simulink model "CW_M107"  (R2017b)
settings: Solver=VariableStepAuto  StartTime=0.0  StopTime=10.0  RelTol=1e-3
undefined symbols (not defined in the file): b, J, K, L, R

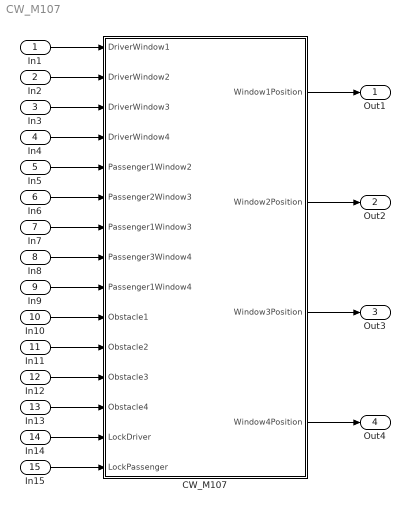
== system CW_M107 ==
  In1 : Inport
  In2 : Inport  Port=2
  In3 : Inport  Port=3
  In4 : Inport  Port=4
  In5 : Inport  Port=5
  In6 : Inport  Port=6
  In7 : Inport  Port=7
  In8 : Inport  Port=8
  In9 : Inport  Port=9
  In10 : Inport  Port=10
  In11 : Inport  Port=11
  In12 : Inport  Port=12
  In13 : Inport  Port=13
  In14 : Inport  Port=14
  In15 : Inport  Port=15
  CW_M107 : Subsystem
  Out1 : Outport
  Out2 : Outport  Port=2
  Out3 : Outport  Port=3
  Out4 : Outport  Port=4
  wires:
  In13/1 -> CW_M107/13(Obstacle4)
  In6/1 -> CW_M107/6(Passenger2Window3)
  CW_M107/2(Window2Position) -> Out2/1
  In9/1 -> CW_M107/9(Passenger1Window4)
  In7/1 -> CW_M107/7(Passenger1Window3)
  In1/1 -> CW_M107/1(DriverWindow1)
  CW_M107/3(Window3Position) -> Out3/1
  In3/1 -> CW_M107/3(DriverWindow3)
  In8/1 -> CW_M107/8(Passenger3Window4)
  CW_M107/4(Window4Position) -> Out4/1
  In15/1 -> CW_M107/15(LockPassenger)
  In5/1 -> CW_M107/5(Passenger1Window2)
  In4/1 -> CW_M107/4(DriverWindow4)
  In10/1 -> CW_M107/10(Obstacle1)
  In14/1 -> CW_M107/14(LockDriver)
  In11/1 -> CW_M107/11(Obstacle2)
  In12/1 -> CW_M107/12(Obstacle3)
  In2/1 -> CW_M107/2(DriverWindow2)
  CW_M107/1(Window1Position) -> Out1/1

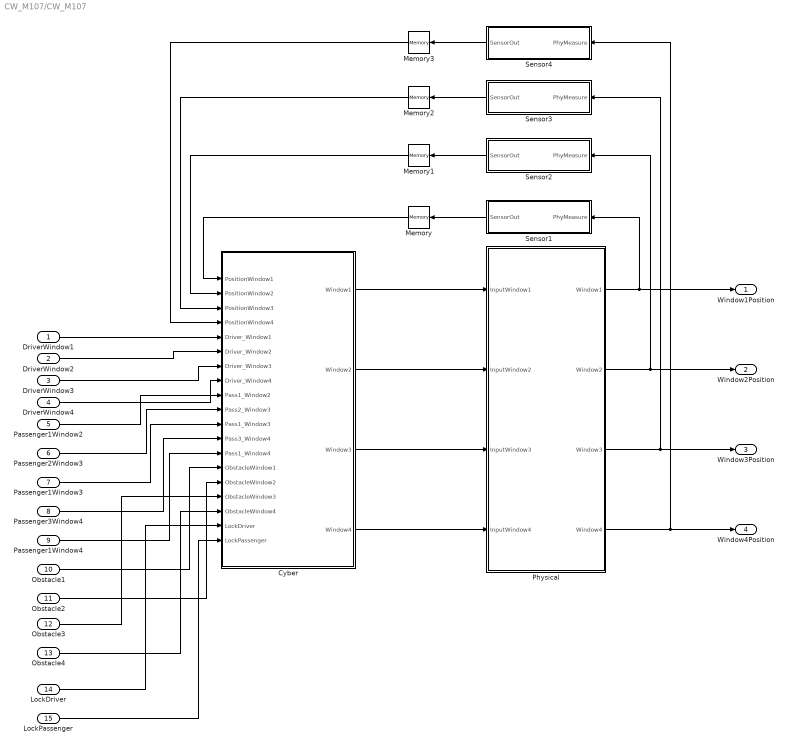
== system CW_M107/CW_M107 ==
  DriverWindow1 : Inport
  DriverWindow2 : Inport  Port=2
  DriverWindow3 : Inport  Port=3
  DriverWindow4 : Inport  Port=4
  Passenger1Window2 : Inport  Port=5
  Passenger2Window3 : Inport  Port=6
  Passenger1Window3 : Inport  Port=7
  Passenger3Window4 : Inport  Port=8
  Passenger1Window4 : Inport  Port=9
  Obstacle1 : Inport  Port=10
  Obstacle2 : Inport  Port=11
  Obstacle3 : Inport  Port=12
  Obstacle4 : Inport  Port=13
  LockDriver : Inport  Port=14
  LockPassenger : Inport  Port=15
  Cyber : Subsystem
  Memory{,1..3} (4 alike) : Memory
  Physical : Subsystem
  Sensor1 : Subsystem
  Sensor2 : Subsystem
  Sensor3 : Subsystem
  Sensor4 : Subsystem
  Window1Position : Outport
  Window2Position : Outport  Port=2
  Window3Position : Outport  Port=3
  Window4Position : Outport  Port=4
  wires:
  LockPassenger/1 -> Cyber/19(LockPassenger)
  LockDriver/1 -> Cyber/18(LockDriver)
  Obstacle4/1 -> Cyber/17(ObstacleWindow4)
  Obstacle3/1 -> Cyber/16(ObstacleWindow3)
  Obstacle2/1 -> Cyber/15(ObstacleWindow2)
  Passenger1Window4/1 -> Cyber/13(Pass1_Window4)
  Passenger3Window4/1 -> Cyber/12(Pass3_Window4)
  Passenger1Window3/1 -> Cyber/11(Pass1_Window3)
  Passenger2Window3/1 -> Cyber/10(Pass2_Window3)
  Passenger1Window2/1 -> Cyber/9(Pass1_Window2)
  DriverWindow4/1 -> Cyber/8(Driver_Window4)
  DriverWindow3/1 -> Cyber/7(Driver_Window3)
  DriverWindow1/1 -> Cyber/5(Driver_Window1)
  DriverWindow2/1 -> Cyber/6(Driver_Window2)
  Sensor1/1(SensorOut) -> Memory/1
  Sensor2/1(SensorOut) -> Memory1/1
  Sensor3/1(SensorOut) -> Memory2/1
  Sensor4/1(SensorOut) -> Memory3/1
  Obstacle1/1 -> Cyber/14(ObstacleWindow1)
  Memory3/1 -> Cyber/4(PositionWindow4)
  Memory2/1 -> Cyber/3(PositionWindow3)
  Memory1/1 -> Cyber/2(PositionWindow2)
  Memory/1 -> Cyber/1(PositionWindow1)
  Physical/4(Window4) -> Window4Position/1, Sensor4/1(PhyMeasure)
  Physical/3(Window3) -> Sensor3/1(PhyMeasure), Window3Position/1
  Physical/2(Window2) -> Window2Position/1, Sensor2/1(PhyMeasure)
  Physical/1(Window1) -> Window1Position/1, Sensor1/1(PhyMeasure)
  Cyber/1(Window1) -> Physical/1(InputWindow1)
  Cyber/2(Window2) -> Physical/2(InputWindow2)
  Cyber/3(Window3) -> Physical/3(InputWindow3)
  Cyber/4(Window4) -> Physical/4(InputWindow4)

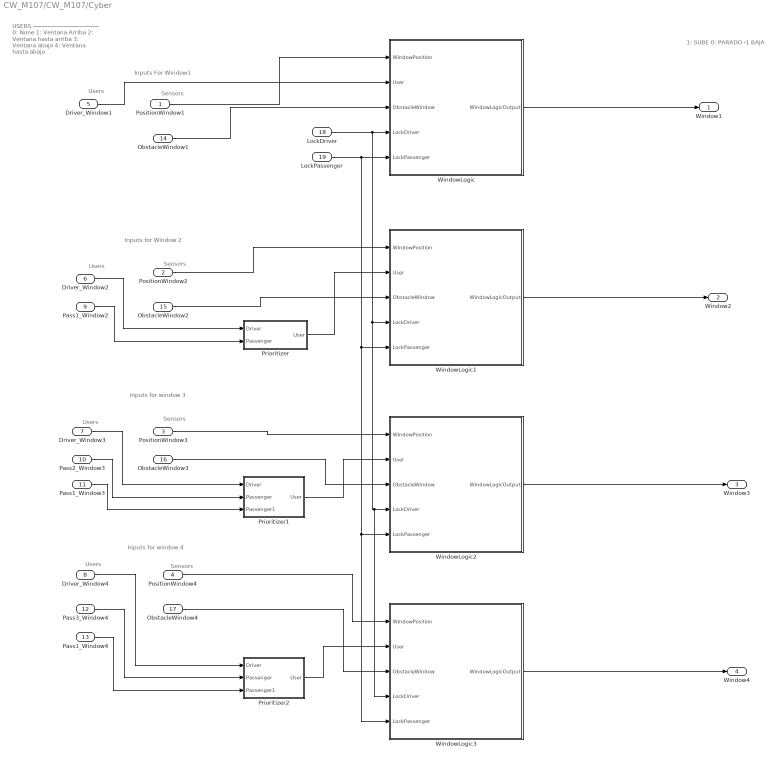
== system CW_M107/CW_M107/Cyber ==
  note: Inputs For Window1
  note: Inputs for Window 2
  note: Inputs for window 3
  note: Inputs for window 4
  note: Sensors
  note: Users
  note: Users
  note: Sensors
  note: Users
  note: Sensors
  note: Users
  note: Sensors
  note: USERS
      | ---------------------------------
      | 0: None
      | 1: Ventana Arriba
      | 2: Ventana hasta arriba
      | 3: Ventana abajo
      | 4: Ventana hasta abajo
  note: 1: SUBE
      | 0: PARADO
      | -1 BAJA
  PositionWindow1 : Inport
  PositionWindow2 : Inport  Port=2
  PositionWindow3 : Inport  Port=3
  PositionWindow4 : Inport  Port=4
  Driver_Window1 : Inport  Port=5
  Driver_Window2 : Inport  Port=6
  Driver_Window3 : Inport  Port=7
  Driver_Window4 : Inport  Port=8
  Pass1_Window2 : Inport  Port=9
  Pass2_Window3 : Inport  Port=10
  Pass1_Window3 : Inport  Port=11
  Pass3_Window4 : Inport  Port=12
  Pass1_Window4 : Inport  Port=13
  ObstacleWindow1 : Inport  Port=14
  ObstacleWindow2 : Inport  Port=15
  ObstacleWindow3 : Inport  Port=16
  ObstacleWindow4 : Inport  Port=17
  LockDriver : Inport  Port=18
  LockPassenger : Inport  Port=19
  Prioritizer : Subsystem
  Prioritizer1 : Subsystem
  Prioritizer2 : Subsystem
  WindowLogic : Subsystem
  WindowLogic1 : Subsystem
  WindowLogic2 : Subsystem
  WindowLogic3 : Subsystem
  Window1 : Outport
  Window2 : Outport  Port=2
  Window3 : Outport  Port=3
  Window4 : Outport  Port=4
  wires:
  WindowLogic3/1(WindowLogicOutput) -> Window4/1
  WindowLogic2/1(WindowLogicOutput) -> Window3/1
  Prioritizer2/1(User) -> WindowLogic3/2(User)
  ObstacleWindow4/1 -> WindowLogic3/3(ObstacleWindow)
  PositionWindow4/1 -> WindowLogic3/1(WindowPosition)
  Pass1_Window4/1 -> Prioritizer2/3(Passenger1)
  Pass3_Window4/1 -> Prioritizer2/2(Passenger)
  Driver_Window4/1 -> Prioritizer2/1(Driver)
  Pass1_Window3/1 -> Prioritizer1/3(Passenger1)
  Pass2_Window3/1 -> Prioritizer1/2(Passenger)
  Driver_Window3/1 -> Prioritizer1/1(Driver)
  ObstacleWindow3/1 -> WindowLogic2/3(ObstacleWindow)
  PositionWindow3/1 -> WindowLogic2/1(WindowPosition)
  Prioritizer1/1(User) -> WindowLogic2/2(User)
  WindowLogic1/1(WindowLogicOutput) -> Window2/1
  ObstacleWindow2/1 -> WindowLogic1/3(ObstacleWindow)
  PositionWindow2/1 -> WindowLogic1/1(WindowPosition)
  Pass1_Window2/1 -> Prioritizer/2(Passenger)
  Driver_Window2/1 -> Prioritizer/1(Driver)
  Prioritizer/1(User) -> WindowLogic1/2(User)
  WindowLogic/1(WindowLogicOutput) -> Window1/1
  Driver_Window1/1 -> WindowLogic/2(User)
  ObstacleWindow1/1 -> WindowLogic/3(ObstacleWindow)
  PositionWindow1/1 -> WindowLogic/1(WindowPosition)
  LockPassenger/1 -> WindowLogic/5(LockPassenger), WindowLogic2/5(LockPassenger), WindowLogic3/5(LockPassenger), WindowLogic1/5(LockPassenger)
  LockDriver/1 -> WindowLogic/4(LockDriver), WindowLogic2/4(LockDriver), WindowLogic3/4(LockDriver), WindowLogic1/4(LockDriver)

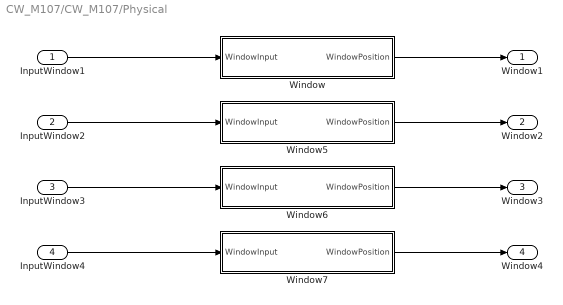
== system CW_M107/CW_M107/Physical ==
  InputWindow1 : Inport
  InputWindow2 : Inport  Port=2
  InputWindow3 : Inport  Port=3
  InputWindow4 : Inport  Port=4
  Window : Subsystem
  Window5 : Subsystem
  Window6 : Subsystem
  Window7 : Subsystem
  Window1 : Outport
  Window2 : Outport  Port=2
  Window3 : Outport  Port=3
  Window4 : Outport  Port=4
  wires:
  Window7/1(WindowPosition) -> Window4/1
  Window6/1(WindowPosition) -> Window3/1
  Window5/1(WindowPosition) -> Window2/1
  Window/1(WindowPosition) -> Window1/1
  InputWindow4/1 -> Window7/1(WindowInput)
  InputWindow3/1 -> Window6/1(WindowInput)
  InputWindow2/1 -> Window5/1(WindowInput)
  InputWindow1/1 -> Window/1(WindowInput)

== system CW_M107/CW_M107/Sensor1 ==
  PhyMeasure : Inport
  SensorOut : Outport
  wires:
  PhyMeasure/1 -> SensorOut/1

== system CW_M107/CW_M107/Sensor2 ==
  PhyMeasure : Inport
  SensorOut : Outport
  wires:
  PhyMeasure/1 -> SensorOut/1

== system CW_M107/CW_M107/Sensor3 ==
  PhyMeasure : Inport
  SensorOut : Outport
  wires:
  PhyMeasure/1 -> SensorOut/1

== system CW_M107/CW_M107/Sensor4 ==
  PhyMeasure : Inport
  SensorOut : Outport
  wires:
  PhyMeasure/1 -> SensorOut/1

== system CW_M107/CW_M107/Cyber/Prioritizer ==
  Driver : Inport
  Passenger : Inport  Port=2
  Switch : Switch  Criteria=u2 ~= 0
  User : Outport
  wires:
  Switch/1 -> User/1
  Passenger/1 -> Switch/3
  Driver/1 -> Switch/2, Switch/1

== system CW_M107/CW_M107/Cyber/Prioritizer1 ==
  Driver : Inport
  Passenger : Inport  Port=2
  Passenger1 : Inport  Port=3
  Switch : Switch  Criteria=u2 ~= 0
  Switch1 : Switch  Criteria=u2 ~= 0
  User : Outport
  wires:
  Switch1/1 -> Switch/3
  Passenger1/1 -> Switch1/3
  Driver/1 -> Switch/2, Switch/1
  Passenger/1 -> Switch1/2, Switch1/1
  Switch/1 -> User/1

== system CW_M107/CW_M107/Cyber/Prioritizer2 ==
  Driver : Inport
  Passenger : Inport  Port=2
  Passenger1 : Inport  Port=3
  Switch : Switch  Criteria=u2 ~= 0
  Switch1 : Switch  Criteria=u2 ~= 0
  User : Outport
  wires:
  Switch/1 -> User/1
  Passenger/1 -> Switch1/1, Switch1/2
  Driver/1 -> Switch/1, Switch/2
  Passenger1/1 -> Switch1/3
  Switch1/1 -> Switch/3

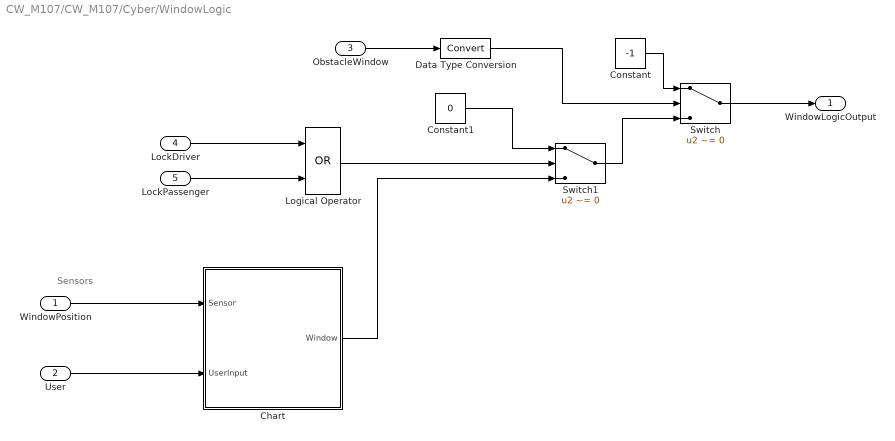
== system CW_M107/CW_M107/Cyber/WindowLogic ==
  note: Sensors
  WindowPosition : Inport
  User : Inport  Port=2
  ObstacleWindow : Inport  Port=3
  LockDriver : Inport  Port=4
  LockPassenger : Inport  Port=5
  Chart : Stateflow chart  TreatAsAtomicUnit=on
  Constant : Constant  Value=-1
  Constant1 : Constant  Value=0
  Data Type Conversion : DataTypeConversion
  Logical Operator : Logic  Operator=OR  AllPortsSameDT=off  OutDataTypeStr=boolean
  Switch : Switch  Criteria=u2 ~= 0  Threshold=1  ZeroCross=off
  Switch1 : Switch  Criteria=u2 ~= 0
  WindowLogicOutput : Outport
  wires:
  Logical Operator/1 -> Switch1/2
  Data Type Conversion/1 -> Switch/2
  Constant/1 -> Switch/1
  Chart/1(Window) -> Switch1/3
  User/1 -> Chart/2(UserInput)
  WindowPosition/1 -> Chart/1(Sensor)
  Switch1/1 -> Switch/3
  Constant1/1 -> Switch1/1
  Switch/1 -> WindowLogicOutput/1
  ObstacleWindow/1 -> Data Type Conversion/1
  LockPassenger/1 -> Logical Operator/2
  LockDriver/1 -> Logical Operator/1

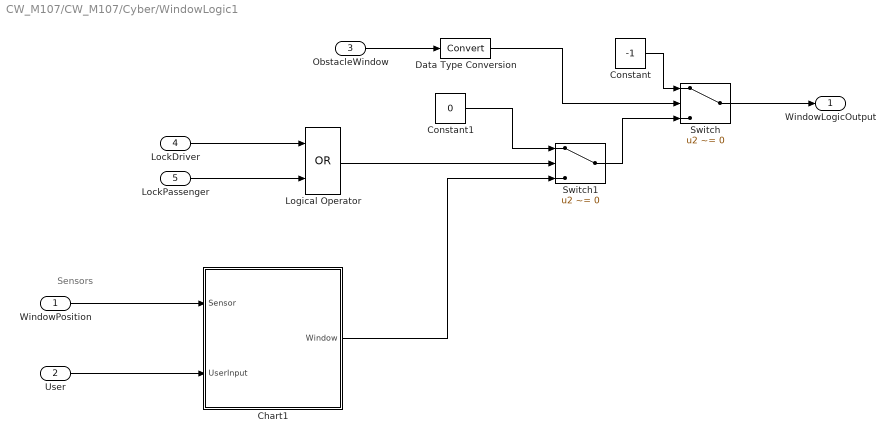
== system CW_M107/CW_M107/Cyber/WindowLogic1 ==
  note: Sensors
  WindowPosition : Inport
  User : Inport  Port=2
  ObstacleWindow : Inport  Port=3
  LockDriver : Inport  Port=4
  LockPassenger : Inport  Port=5
  Chart1 : Stateflow chart  TreatAsAtomicUnit=on
  Constant : Constant  Value=-1
  Constant1 : Constant  Value=0
  Data Type Conversion : DataTypeConversion
  Logical Operator : Logic  Operator=OR  AllPortsSameDT=off  OutDataTypeStr=boolean
  Switch : Switch  Criteria=u2 ~= 0  Threshold=1  ZeroCross=off
  Switch1 : Switch  Criteria=u2 ~= 0
  WindowLogicOutput : Outport
  wires:
  LockDriver/1 -> Logical Operator/1
  LockPassenger/1 -> Logical Operator/2
  ObstacleWindow/1 -> Data Type Conversion/1
  Switch/1 -> WindowLogicOutput/1
  Constant1/1 -> Switch1/1
  Switch1/1 -> Switch/3
  WindowPosition/1 -> Chart1/1(Sensor)
  User/1 -> Chart1/2(UserInput)
  Chart1/1(Window) -> Switch1/3
  Constant/1 -> Switch/1
  Data Type Conversion/1 -> Switch/2
  Logical Operator/1 -> Switch1/2

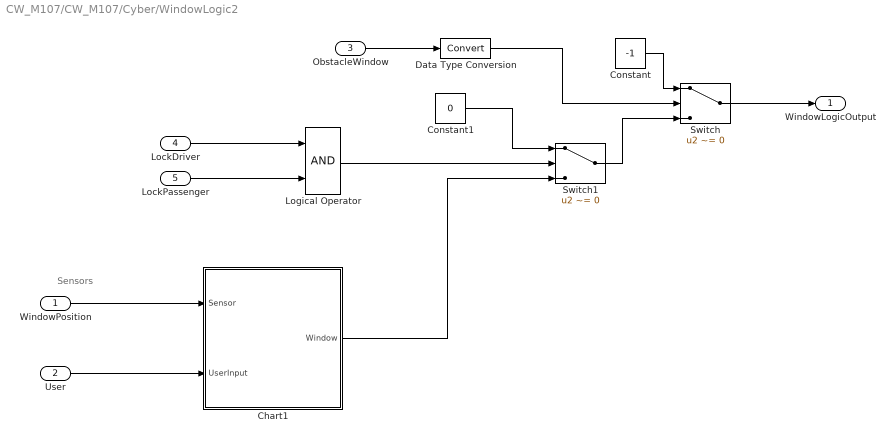
== system CW_M107/CW_M107/Cyber/WindowLogic2 ==
  note: Sensors
  WindowPosition : Inport
  User : Inport  Port=2
  ObstacleWindow : Inport  Port=3
  LockDriver : Inport  Port=4
  LockPassenger : Inport  Port=5
  Chart1 : Stateflow chart  TreatAsAtomicUnit=on
  Constant : Constant  Value=-1
  Constant1 : Constant  Value=0
  Data Type Conversion : DataTypeConversion
  Logical Operator : Logic  AllPortsSameDT=off  OutDataTypeStr=boolean
  Switch : Switch  Criteria=u2 ~= 0  Threshold=1  ZeroCross=off
  Switch1 : Switch  Criteria=u2 ~= 0
  WindowLogicOutput : Outport
  wires:
  Logical Operator/1 -> Switch1/2
  Data Type Conversion/1 -> Switch/2
  Constant/1 -> Switch/1
  Chart1/1(Window) -> Switch1/3
  User/1 -> Chart1/2(UserInput)
  WindowPosition/1 -> Chart1/1(Sensor)
  Switch1/1 -> Switch/3
  Constant1/1 -> Switch1/1
  Switch/1 -> WindowLogicOutput/1
  ObstacleWindow/1 -> Data Type Conversion/1
  LockPassenger/1 -> Logical Operator/2
  LockDriver/1 -> Logical Operator/1

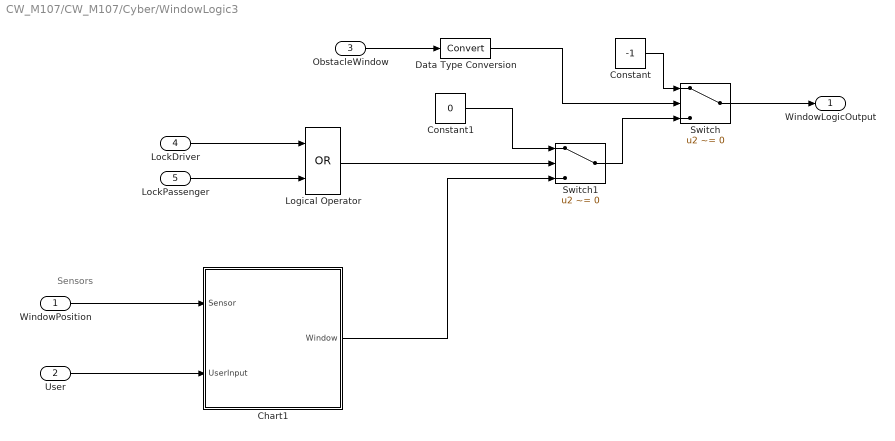
== system CW_M107/CW_M107/Cyber/WindowLogic3 ==
  note: Sensors
  WindowPosition : Inport
  User : Inport  Port=2
  ObstacleWindow : Inport  Port=3
  LockDriver : Inport  Port=4
  LockPassenger : Inport  Port=5
  Chart1 : Stateflow chart  TreatAsAtomicUnit=on
  Constant : Constant  Value=-1
  Constant1 : Constant  Value=0
  Data Type Conversion : DataTypeConversion
  Logical Operator : Logic  Operator=OR  AllPortsSameDT=off  OutDataTypeStr=boolean
  Switch : Switch  Criteria=u2 ~= 0  Threshold=1  ZeroCross=off
  Switch1 : Switch  Criteria=u2 ~= 0
  WindowLogicOutput : Outport
  wires:
  LockDriver/1 -> Logical Operator/1
  LockPassenger/1 -> Logical Operator/2
  ObstacleWindow/1 -> Data Type Conversion/1
  Switch/1 -> WindowLogicOutput/1
  Constant1/1 -> Switch1/1
  Switch1/1 -> Switch/3
  WindowPosition/1 -> Chart1/1(Sensor)
  User/1 -> Chart1/2(UserInput)
  Chart1/1(Window) -> Switch1/3
  Constant/1 -> Switch/1
  Data Type Conversion/1 -> Switch/2
  Logical Operator/1 -> Switch1/2

== system CW_M107/CW_M107/Physical/Window ==
  WindowInput : Inport
  DC_Engine : Subsystem
  Integrator : Integrator  InitialCondition=5  LimitOutput=on  UpperSaturationLimit=5  LowerSaturationLimit=0
  WindowPosition : Outport
  wires:
  WindowInput/1 -> DC_Engine/1(input)
  DC_Engine/1(Speed) -> Integrator/1
  Integrator/1 -> WindowPosition/1

== system CW_M107/CW_M107/Physical/Window5 ==
  WindowInput : Inport
  DC_Engine : Subsystem
  Integrator : Integrator  InitialCondition=5  LimitOutput=on  UpperSaturationLimit=5  LowerSaturationLimit=0
  WindowPosition : Outport
  wires:
  Integrator/1 -> WindowPosition/1
  DC_Engine/1(Speed) -> Integrator/1
  WindowInput/1 -> DC_Engine/1(input)

== system CW_M107/CW_M107/Physical/Window6 ==
  WindowInput : Inport
  DC_Engine : Subsystem
  Integrator : Integrator  InitialCondition=5  LimitOutput=on  UpperSaturationLimit=5  LowerSaturationLimit=0
  WindowPosition : Outport
  wires:
  WindowInput/1 -> DC_Engine/1(input)
  DC_Engine/1(Speed) -> Integrator/1
  Integrator/1 -> WindowPosition/1

== system CW_M107/CW_M107/Physical/Window7 ==
  WindowInput : Inport
  DC_Engine : Subsystem
  Integrator : Integrator  InitialCondition=5  LimitOutput=on  UpperSaturationLimit=5  LowerSaturationLimit=0
  WindowPosition : Outport
  wires:
  Integrator/1 -> WindowPosition/1
  DC_Engine/1(Speed) -> Integrator/1
  WindowInput/1 -> DC_Engine/1(input)

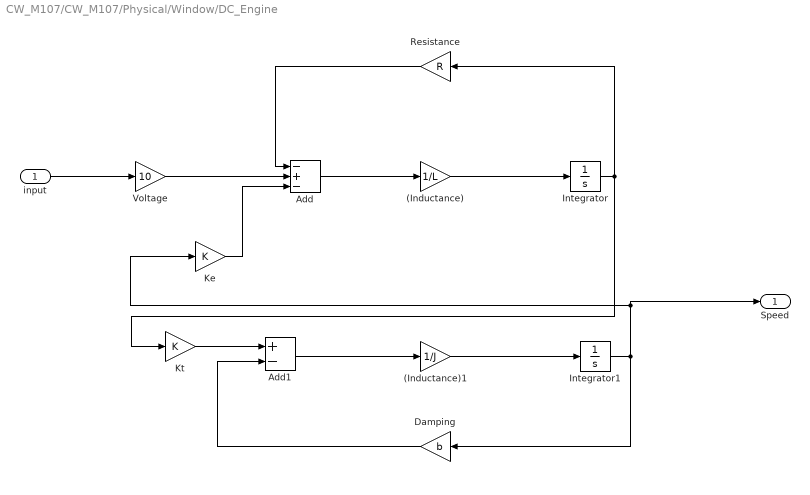
== system CW_M107/CW_M107/Physical/Window/DC_Engine ==
  input : Inport
  (Inductance) : Gain  Gain=1/L
  (Inductance)1 : Gain  Gain=1/J
  Add : Sum  Inputs=-+-
  Add1 : Sum  Inputs=+-
  Damping : Gain  Gain=b
  Integrator : Integrator
  Integrator1 : Integrator
  Ke : Gain  Gain=K
  Kt : Gain  Gain=K
  Resistance : Gain  Gain=R
  Voltage : Gain  Gain=10
  Speed : Outport
  wires:
  Damping/1 -> Add1/2
  Integrator1/1 -> Damping/1, Speed/1, Ke/1
  (Inductance)1/1 -> Integrator1/1
  Add1/1 -> (Inductance)1/1
  Kt/1 -> Add1/1
  Ke/1 -> Add/3
  Resistance/1 -> Add/1
  Integrator/1 -> Resistance/1, Kt/1
  (Inductance)/1 -> Integrator/1
  Add/1 -> (Inductance)/1
  Voltage/1 -> Add/2
  input/1 -> Voltage/1

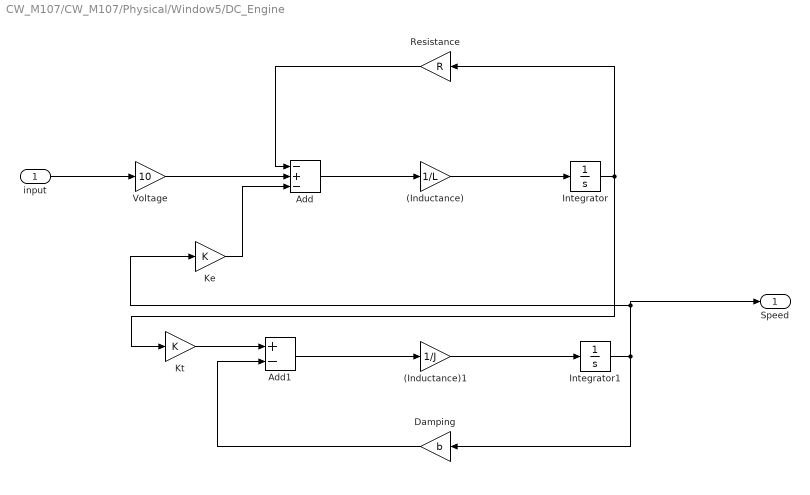
== system CW_M107/CW_M107/Physical/Window5/DC_Engine ==
  input : Inport
  (Inductance) : Gain  Gain=1/L
  (Inductance)1 : Gain  Gain=1/J
  Add : Sum  Inputs=-+-
  Add1 : Sum  Inputs=+-
  Damping : Gain  Gain=b
  Integrator : Integrator
  Integrator1 : Integrator
  Ke : Gain  Gain=K
  Kt : Gain  Gain=K
  Resistance : Gain  Gain=R
  Voltage : Gain  Gain=10
  Speed : Outport
  wires:
  input/1 -> Voltage/1
  Voltage/1 -> Add/2
  Add/1 -> (Inductance)/1
  (Inductance)/1 -> Integrator/1
  Integrator/1 -> Kt/1, Resistance/1
  Resistance/1 -> Add/1
  Ke/1 -> Add/3
  Kt/1 -> Add1/1
  Add1/1 -> (Inductance)1/1
  (Inductance)1/1 -> Integrator1/1
  Integrator1/1 -> Ke/1, Speed/1, Damping/1
  Damping/1 -> Add1/2

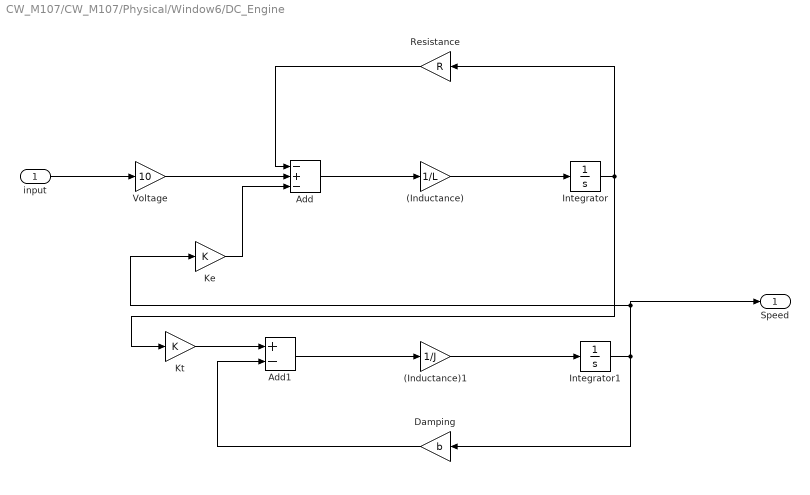
== system CW_M107/CW_M107/Physical/Window6/DC_Engine ==
  input : Inport
  (Inductance) : Gain  Gain=1/L
  (Inductance)1 : Gain  Gain=1/J
  Add : Sum  Inputs=-+-
  Add1 : Sum  Inputs=+-
  Damping : Gain  Gain=b
  Integrator : Integrator
  Integrator1 : Integrator
  Ke : Gain  Gain=K
  Kt : Gain  Gain=K
  Resistance : Gain  Gain=R
  Voltage : Gain  Gain=10
  Speed : Outport
  wires:
  Damping/1 -> Add1/2
  Integrator1/1 -> Damping/1, Speed/1, Ke/1
  (Inductance)1/1 -> Integrator1/1
  Add1/1 -> (Inductance)1/1
  Kt/1 -> Add1/1
  Ke/1 -> Add/3
  Resistance/1 -> Add/1
  Integrator/1 -> Resistance/1, Kt/1
  (Inductance)/1 -> Integrator/1
  Add/1 -> (Inductance)/1
  Voltage/1 -> Add/2
  input/1 -> Voltage/1

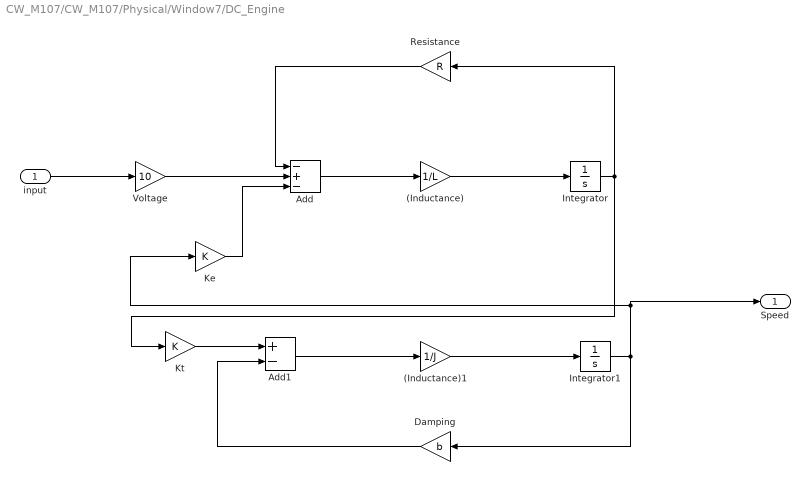
== system CW_M107/CW_M107/Physical/Window7/DC_Engine ==
  input : Inport
  (Inductance) : Gain  Gain=1/L
  (Inductance)1 : Gain  Gain=1/J
  Add : Sum  Inputs=-+-
  Add1 : Sum  Inputs=+-
  Damping : Gain  Gain=b
  Integrator : Integrator
  Integrator1 : Integrator
  Ke : Gain  Gain=K
  Kt : Gain  Gain=K
  Resistance : Gain  Gain=R
  Voltage : Gain  Gain=10
  Speed : Outport
  wires:
  input/1 -> Voltage/1
  Voltage/1 -> Add/2
  Add/1 -> (Inductance)/1
  (Inductance)/1 -> Integrator/1
  Integrator/1 -> Kt/1, Resistance/1
  Resistance/1 -> Add/1
  Ke/1 -> Add/3
  Kt/1 -> Add1/1
  Add1/1 -> (Inductance)1/1
  (Inductance)1/1 -> Integrator1/1
  Integrator1/1 -> Ke/1, Speed/1, Damping/1
  Damping/1 -> Add1/2

== stateflow chart CW_M107/Cyber/WindowLogic/Chart ==
  state Bajand_hasta_abajo
    entry: Window = -1;
  state Bajando
    entry: Window = -1;
  state Idle
    entry:Window = 0;
  state Subiendo_hasta_arriba
    entry: Window = 1;
  state Subiendo
    entry: Window = 1;
  Subiendo -> Bajand_hasta_abajo [order 4] : [UserInput==4]
  Bajand_hasta_abajo -> Bajando [order 2] : [UserInput==3]
  Subiendo -> Bajando [order 3] : [UserInput==3]
  Bajando -> Bajand_hasta_abajo [order 2] : [UserInput==4]
  Idle -> Bajando [order 3] : [UserInput==3&&Sensor>0]
  Subiendo_hasta_arriba -> Bajand_hasta_abajo [order 3] : [UserInput==4]
  Idle -> Bajand_hasta_abajo [order 4] : [UserInput==4&&Sensor>0]
  Bajando -> Subiendo [order 3] : [UserInput==1]
  Subiendo_hasta_arriba -> Bajando [order 4] : [UserInput==3]
  Bajand_hasta_abajo -> Subiendo [order 4] : [UserInput==1]
  Bajand_hasta_abajo -> Idle [order 1] : [Sensor<=0]
  Bajand_hasta_abajo -> Subiendo_hasta_arriba [order 3] : [UserInput==2]
  Bajando -> Idle [order 1] : [Sensor<=0||UserInput==0]
  Bajando -> Subiendo_hasta_arriba [order 4] : [UserInput==2]
  (default) -> Idle
  Idle -> Subiendo_hasta_arriba [order 2] : [UserInput==2&&Sensor<5]
  Idle -> Subiendo [order 1] : [UserInput == 1&&Sensor<5]
  Subiendo -> Idle [order 1] : [Sensor>=5||UserInput==0]
  Subiendo_hasta_arriba -> Idle [order 1] : [Sensor >=5]
  Subiendo_hasta_arriba -> Subiendo [order 2] : [UserInput ==1]
  Subiendo -> Subiendo_hasta_arriba [order 2] : [UserInput==2]
  data: Sensor input; UserInput input; Window output double

== stateflow chart CW_M107/Cyber/WindowLogic1/Chart1 ==
  state Bajand_hasta_abajo
    entry: Window = -1;
  state Bajando
    entry: Window = -1;
  state Idle
    entry:Window = 0;
  state Subiendo_hasta_arriba
    entry: Window = 1;
  state Subiendo
    entry: Window = 1;
  Subiendo -> Bajand_hasta_abajo [order 4] : [UserInput==4]
  Bajand_hasta_abajo -> Bajando [order 2] : [UserInput==3]
  Subiendo -> Bajando [order 3] : [UserInput==3]
  Bajando -> Bajand_hasta_abajo [order 2] : [UserInput==4]
  Idle -> Bajando [order 3] : [UserInput==3&&Sensor>0]
  Subiendo_hasta_arriba -> Bajand_hasta_abajo [order 3] : [UserInput==4]
  Idle -> Bajand_hasta_abajo [order 4] : [UserInput==4&&Sensor>0]
  Bajando -> Subiendo [order 3] : [UserInput==1]
  Subiendo_hasta_arriba -> Bajando [order 4] : [UserInput==3]
  Bajand_hasta_abajo -> Subiendo [order 4] : [UserInput==1]
  Bajand_hasta_abajo -> Idle [order 1] : [Sensor<=0]
  Bajand_hasta_abajo -> Subiendo_hasta_arriba [order 3] : [UserInput==2]
  Bajando -> Idle [order 1] : [Sensor<=0||UserInput==0]
  Bajando -> Subiendo_hasta_arriba [order 4] : [UserInput==2]
  (default) -> Idle
  Idle -> Subiendo_hasta_arriba [order 2] : [UserInput==2&&Sensor<5]
  Idle -> Subiendo [order 1] : [UserInput == 1&&Sensor<5]
  Subiendo -> Idle [order 1] : [Sensor>=5||UserInput==0]
  Subiendo_hasta_arriba -> Idle [order 1] : [Sensor >=5]
  Subiendo_hasta_arriba -> Subiendo [order 2] : [UserInput ==1]
  Subiendo -> Subiendo_hasta_arriba [order 2] : [UserInput==2]
  data: Sensor input; UserInput input; Window output double

== stateflow chart CW_M107/Cyber/WindowLogic2/Chart1 ==
  state Bajand_hasta_abajo
    entry: Window = -1;
  state Bajando
    entry: Window = -1;
  state Idle
    entry:Window = 0;
  state Subiendo_hasta_arriba
    entry: Window = 1;
  state Subiendo
    entry: Window = 1;
  Subiendo -> Bajand_hasta_abajo [order 4] : [UserInput==4]
  Bajand_hasta_abajo -> Bajando [order 2] : [UserInput==3]
  Subiendo -> Bajando [order 3] : [UserInput==3]
  Bajando -> Bajand_hasta_abajo [order 2] : [UserInput==4]
  Idle -> Bajando [order 3] : [UserInput==3&&Sensor>0]
  Subiendo_hasta_arriba -> Bajand_hasta_abajo [order 3] : [UserInput==4]
  Idle -> Bajand_hasta_abajo [order 4] : [UserInput==4&&Sensor>0]
  Bajando -> Subiendo [order 3] : [UserInput==1]
  Subiendo_hasta_arriba -> Bajando [order 4] : [UserInput==3]
  Bajand_hasta_abajo -> Subiendo [order 4] : [UserInput==1]
  Bajand_hasta_abajo -> Idle [order 1] : [Sensor<=0]
  Bajand_hasta_abajo -> Subiendo_hasta_arriba [order 3] : [UserInput==2]
  Bajando -> Idle [order 1] : [Sensor<=0||UserInput==0]
  Bajando -> Subiendo_hasta_arriba [order 4] : [UserInput==2]
  (default) -> Idle
  Idle -> Subiendo_hasta_arriba [order 2] : [UserInput==2&&Sensor<5]
  Idle -> Subiendo [order 1] : [UserInput == 1&&Sensor<5]
  Subiendo -> Idle [order 1] : [Sensor>=5||UserInput==0]
  Subiendo_hasta_arriba -> Idle [order 1] : [Sensor >=5]
  Subiendo_hasta_arriba -> Subiendo [order 2] : [UserInput ==1]
  Subiendo -> Subiendo_hasta_arriba [order 2] : [UserInput==2]
  data: Sensor input; UserInput input; Window output double

== stateflow chart CW_M107/Cyber/WindowLogic3/Chart1 ==
  state Bajand_hasta_abajo
    entry: Window = -1;
  state Bajando
    entry: Window = -1;
  state Idle
    entry:Window = 0;
  state Subiendo_hasta_arriba
    entry: Window = 1;
  state Subiendo
    entry: Window = 1;
  Subiendo -> Bajand_hasta_abajo [order 4] : [UserInput==4]
  Bajand_hasta_abajo -> Bajando [order 2] : [UserInput==3]
  Subiendo -> Bajando [order 3] : [UserInput==3]
  Bajando -> Bajand_hasta_abajo [order 2] : [UserInput==4]
  Idle -> Bajando [order 3] : [UserInput==3&&Sensor>0]
  Subiendo_hasta_arriba -> Bajand_hasta_abajo [order 3] : [UserInput==4]
  Idle -> Bajand_hasta_abajo [order 4] : [UserInput==4&&Sensor>0]
  Bajando -> Subiendo [order 3] : [UserInput==1]
  Subiendo_hasta_arriba -> Bajando [order 4] : [UserInput==3]
  Bajand_hasta_abajo -> Subiendo [order 4] : [UserInput==1]
  Bajand_hasta_abajo -> Idle [order 1] : [Sensor<=0]
  Bajand_hasta_abajo -> Subiendo_hasta_arriba [order 3] : [UserInput==2]
  Bajando -> Idle [order 1] : [Sensor<=0||UserInput==0]
  Bajando -> Subiendo_hasta_arriba [order 4] : [UserInput==2]
  (default) -> Idle
  Idle -> Subiendo_hasta_arriba [order 2] : [UserInput==2&&Sensor<5]
  Idle -> Subiendo [order 1] : [UserInput == 1&&Sensor<5]
  Subiendo -> Idle [order 1] : [Sensor>=5||UserInput==0]
  Subiendo_hasta_arriba -> Idle [order 1] : [Sensor >=5]
  Subiendo_hasta_arriba -> Subiendo [order 2] : [UserInput ==1]
  Subiendo -> Subiendo_hasta_arriba [order 2] : [UserInput==2]
  data: Sensor input; UserInput input; Window output double
